simulink library "halin"  (R2021b)
settings: Solver=VariableStepAuto  StartTime=0.0  StopTime=10.0  RelTol=1e-3
undefined symbols (not defined in the file): KHAL_CAN1ABM1E2E_flg, KHAL_CAN1EPB1E2E_flg, KHAL_CAN1EPS1E2E_flg, KHAL_CAN1ESC1E2E_flg, KHAL_CAN1ESC5E2E_flg, KHAL_CAN3BMS1E2E_flg, KHAL_CAN3BMS6E2E_flg, KHAL_CAN3CCU1E2E_flg, KHAL_CAN3CCU2E2E_flg, KHAL_CAN3MCUBF1E2E_flg, KHAL_CAN3MCUBR1E2E_flg, KHAL_CAN3MCUNF1E2E_flg, KHAL_CAN3MCUNR1E2E_flg, KHAL_CAN3Shifter1E2E_flg, KHAL_CAN3Shifter2E2E_flg, KHAL_CAN6FCM2E2E_flg, KHAL_CAN6FCM4E2E_flg, TRUE
libraries: simulink x791, FVT_lib x214, hcu_lib x58
(part 17 of 25)

== system halin/HAL_IN/CAN4/ZONE_FR1 ==
  DT_CAN4_SG_ZONE_FR1 : Inport
  ChargeInletLockSta : Subsystem
  CompProEN : Subsystem
  FLTurnLPErr : Subsystem
  FLTurnLampC : Subsystem
  FLTurnLightWarning : Subsystem
  FRTurnLPErr : Subsystem
  FRTurnLampC : Subsystem
  FRTurnLightWarning : Subsystem
  FWiperAS : Subsystem
  FWiperProtection : Subsystem
  LADBHibeamIndication : Subsystem
  LADBOperationStatus : Subsystem
  LADBWarning : Subsystem
  LAHBWarning : Subsystem
  LDRLWarning : Subsystem
  LLBWarning : Subsystem
  LpositionLampWarning : Subsystem
  RADBHibeamIndication : Subsystem
  RADBOperationStatus : Subsystem
  RADBWarning : Subsystem
  RAHBWarning : Subsystem
  RDRLWarning : Subsystem
  RLBWarning : Subsystem
  RpositionLampWarning : Subsystem
  TrailerCheck : Subsystem
  TrailerModeSta : Subsystem
  ZFRBCMChargerDoorSWSta : Subsystem
  ZFRBCMHRLTurnLPNormalSta : Subsystem
  ZFRBCMHRRTurnLPHNormalSta : Subsystem
  ZFRTHCMCLEVentActYSta : Subsystem
  ZFRTHCMCREVentActYSta : Subsystem
  ZFRTHCMLEVentActYSta : Subsystem
  ZFRTHCMREVentActYSta : Subsystem
  bus_selector : BusSelector  OutputSignals=CAN4_ChargeInletLockSta
  bus_selector1 : BusSelector  OutputSignals=CAN4_CompProEN
  bus_selector10 : BusSelector  OutputSignals=CAN4_LADB_Hibeam_Indication
  bus_selector11 : BusSelector  OutputSignals=CAN4_LADB_Operation_Status
  bus_selector12 : BusSelector  OutputSignals=CAN4_LADB_Warning
  bus_selector13 : BusSelector  OutputSignals=CAN4_LAHB_Warning
  bus_selector14 : BusSelector  OutputSignals=CAN4_LDRL_Warning
  bus_selector15 : BusSelector  OutputSignals=CAN4_LLB_Warning
  bus_selector16 : BusSelector  OutputSignals=CAN4_Lposition_Lamp_Warning
  bus_selector17 : BusSelector  OutputSignals=CAN4_RADB_Hibeam_Indication
  bus_selector18 : BusSelector  OutputSignals=CAN4_RADB_Operation_Status
  bus_selector19 : BusSelector  OutputSignals=CAN4_RADB_Warning
  bus_selector2 : BusSelector  OutputSignals=CAN4_FLTurnLPErr
  bus_selector20 : BusSelector  OutputSignals=CAN4_RAHB_Warning
  bus_selector21 : BusSelector  OutputSignals=CAN4_RDRL_Warning
  bus_selector22 : BusSelector  OutputSignals=CAN4_RLB_Warning
  bus_selector23 : BusSelector  OutputSignals=CAN4_Rposition_Lamp_Warning
  bus_selector24 : BusSelector  OutputSignals=CAN4_TrailerCheck
  bus_selector25 : BusSelector  OutputSignals=CAN4_TrailerModeSta
  bus_selector26 : BusSelector  OutputSignals=CAN4_ZFR_BCM_ChargerDoorSW_Sta
  bus_selector27 : BusSelector  OutputSignals=CAN4_ZFR_BCM_HRLTurnLPNormal_Sta
  bus_selector28 : BusSelector  OutputSignals=CAN4_ZFR_BCM_HRRTurnLPHNormal_Sta
  bus_selector29 : BusSelector  OutputSignals=CAN4_ZFR_THCM_CLEVentActY_Sta
  bus_selector3 : BusSelector  OutputSignals=CAN4_FLTurnLampC
  bus_selector30 : BusSelector  OutputSignals=CAN4_ZFR_THCM_CREVentActY_Sta
  bus_selector31 : BusSelector  OutputSignals=CAN4_ZFR_THCM_LEVentActY_Sta
  bus_selector32 : BusSelector  OutputSignals=CAN4_ZFR_THCM_REVentActY_Sta
  bus_selector4 : BusSelector  OutputSignals=CAN4_FLTurn_Light_Warning
  bus_selector5 : BusSelector  OutputSignals=CAN4_FRTurnLPErr
  bus_selector6 : BusSelector  OutputSignals=CAN4_FRTurnLampC
  bus_selector7 : BusSelector  OutputSignals=CAN4_FRTurn_Light_Warning
  bus_selector8 : BusSelector  OutputSignals=CAN4_FWiperAS
  bus_selector9 : BusSelector  OutputSignals=CAN4_FWiperProtection
  VHAL_ChargeInletLockSta_flg : Outport
  VHAL_CompProEN_flg : Outport  Port=2
  VHAL_FLTurnLPErr_flg : Outport  Port=3
  VHAL_FLTurnLampC_mA : Outport  Port=4
  VHAL_FLTurnLightWarning_flg : Outport  Port=5
  VHAL_FRTurnLPErr_flg : Outport  Port=6
  VHAL_FRTurnLampC_mA : Outport  Port=7
  VHAL_FRTurnLightWarning_flg : Outport  Port=8
  VHAL_FWiperAS_flg : Outport  Port=9
  VHAL_FWiperProtection_flg : Outport  Port=10
  VHAL_LADBHibeamIndication_flg : Outport  Port=11
  VHAL_LADBOperationStatus_flg : Outport  Port=12
  VHAL_LADBWarning_flg : Outport  Port=13
  VHAL_LAHBWarning_flg : Outport  Port=14
  VHAL_LDRLWarning_flg : Outport  Port=15
  VHAL_LLBWarning_flg : Outport  Port=16
  VHAL_LpositionLampWarning_flg : Outport  Port=17
  VHAL_RADBHibeamIndication_flg : Outport  Port=18
  VHAL_RADBOperationStatus_flg : Outport  Port=19
  VHAL_RADBWarning_flg : Outport  Port=20
  VHAL_RAHBWarning_flg : Outport  Port=21
  VHAL_RDRLWarning_flg : Outport  Port=22
  VHAL_RLBWarning_flg : Outport  Port=23
  VHAL_RpositionLampWarning_flg : Outport  Port=24
  VHAL_TrailerCheck_flg : Outport  Port=25
  VHAL_TrailerModeSta_enum : Outport  Port=26
  VHAL_ZFRBCMChargerDoorSWSta_flg : Outport  Port=27
  VHAL_ZFRBCMHRLTurnLPNormalSta_flg : Outport  Port=28
  VHAL_ZFRBCMHRRTurnLPHNormalSta_flg : Outport  Port=29
  VHAL_ZFRTHCMCLEVentActYSta_pct : Outport  Port=30
  VHAL_ZFRTHCMCREVentActYSta_pct : Outport  Port=31
  VHAL_ZFRTHCMLEVentActYSta_pct : Outport  Port=32
  VHAL_ZFRTHCMREVentActYSta_pct : Outport  Port=33
  wires:
  DT_CAN4_SG_ZONE_FR1/1 -> [DT_CAN4_SG_ZONE_FR1]
  [DT_CAN4_SG_ZONE_FR1] -> bus_selector/1
  bus_selector/1 -> ChargeInletLockSta/1(ChargeInletLockSta)  "<CAN4_ChargeInletLockSta>"
  ChargeInletLockSta/1(VHAL_ChargeInletLockSta_flg) -> VHAL_ChargeInletLockSta_flg/1
  [DT_CAN4_SG_ZONE_FR1] -> bus_selector1/1
  bus_selector1/1 -> CompProEN/1(CompProEN)  "<CAN4_CompProEN>"
  CompProEN/1(VHAL_CompProEN_flg) -> VHAL_CompProEN_flg/1
  [DT_CAN4_SG_ZONE_FR1] -> bus_selector2/1
  bus_selector2/1 -> FLTurnLPErr/1(FLTurnLPErr)  "<CAN4_FLTurnLPErr>"
  FLTurnLPErr/1(VHAL_FLTurnLPErr_flg) -> VHAL_FLTurnLPErr_flg/1
  [DT_CAN4_SG_ZONE_FR1] -> bus_selector3/1
  bus_selector3/1 -> FLTurnLampC/1(FLTurnLampC)  "<CAN4_FLTurnLampC>"
  FLTurnLampC/1(VHAL_FLTurnLampC_mA) -> VHAL_FLTurnLampC_mA/1
  [DT_CAN4_SG_ZONE_FR1] -> bus_selector4/1
  bus_selector4/1 -> FLTurnLightWarning/1(FLTurn_Light_Warning)  "<CAN4_FLTurn_Light_Warning>"
  FLTurnLightWarning/1(VHAL_FLTurnLightWarning_flg) -> VHAL_FLTurnLightWarning_flg/1
  [DT_CAN4_SG_ZONE_FR1] -> bus_selector5/1
  bus_selector5/1 -> FRTurnLPErr/1(FRTurnLPErr)  "<CAN4_FRTurnLPErr>"
  FRTurnLPErr/1(VHAL_FRTurnLPErr_flg) -> VHAL_FRTurnLPErr_flg/1
  [DT_CAN4_SG_ZONE_FR1] -> bus_selector6/1
  bus_selector6/1 -> FRTurnLampC/1(FRTurnLampC)  "<CAN4_FRTurnLampC>"
  FRTurnLampC/1(VHAL_FRTurnLampC_mA) -> VHAL_FRTurnLampC_mA/1
  [DT_CAN4_SG_ZONE_FR1] -> bus_selector7/1
  bus_selector7/1 -> FRTurnLightWarning/1(FRTurn_Light_Warning)  "<CAN4_FRTurn_Light_Warning>"
  FRTurnLightWarning/1(VHAL_FRTurnLightWarning_flg) -> VHAL_FRTurnLightWarning_flg/1
  [DT_CAN4_SG_ZONE_FR1] -> bus_selector8/1
  bus_selector8/1 -> FWiperAS/1(FWiperAS)  "<CAN4_FWiperAS>"
  FWiperAS/1(VHAL_FWiperAS_flg) -> VHAL_FWiperAS_flg/1
  [DT_CAN4_SG_ZONE_FR1] -> bus_selector9/1
  bus_selector9/1 -> FWiperProtection/1(FWiperProtection)  "<CAN4_FWiperProtection>"
  FWiperProtection/1(VHAL_FWiperProtection_flg) -> VHAL_FWiperProtection_flg/1
  [DT_CAN4_SG_ZONE_FR1] -> bus_selector10/1
  bus_selector10/1 -> LADBHibeamIndication/1(LADB_Hibeam_Indication)  "<CAN4_LADB_Hibeam_Indication>"
  LADBHibeamIndication/1(VHAL_LADBHibeamIndication_flg) -> VHAL_LADBHibeamIndication_flg/1
  [DT_CAN4_SG_ZONE_FR1] -> bus_selector11/1
  bus_selector11/1 -> LADBOperationStatus/1(LADB_Operation_Status)  "<CAN4_LADB_Operation_Status>"
  LADBOperationStatus/1(VHAL_LADBOperationStatus_flg) -> VHAL_LADBOperationStatus_flg/1
  [DT_CAN4_SG_ZONE_FR1] -> bus_selector12/1
  bus_selector12/1 -> LADBWarning/1(LADB_Warning)  "<CAN4_LADB_Warning>"
  LADBWarning/1(VHAL_LADBWarning_flg) -> VHAL_LADBWarning_flg/1
  [DT_CAN4_SG_ZONE_FR1] -> bus_selector13/1
  bus_selector13/1 -> LAHBWarning/1(LAHB_Warning)  "<CAN4_LAHB_Warning>"
  LAHBWarning/1(VHAL_LAHBWarning_flg) -> VHAL_LAHBWarning_flg/1
  [DT_CAN4_SG_ZONE_FR1] -> bus_selector14/1
  bus_selector14/1 -> LDRLWarning/1(LDRL_Warning)  "<CAN4_LDRL_Warning>"
  LDRLWarning/1(VHAL_LDRLWarning_flg) -> VHAL_LDRLWarning_flg/1
  [DT_CAN4_SG_ZONE_FR1] -> bus_selector15/1
  bus_selector15/1 -> LLBWarning/1(LLB_Warning)  "<CAN4_LLB_Warning>"
  LLBWarning/1(VHAL_LLBWarning_flg) -> VHAL_LLBWarning_flg/1
  [DT_CAN4_SG_ZONE_FR1] -> bus_selector16/1
  bus_selector16/1 -> LpositionLampWarning/1(Lposition_Lamp_Warning)  "<CAN4_Lposition_Lamp_Warning>"
  LpositionLampWarning/1(VHAL_LpositionLampWarning_flg) -> VHAL_LpositionLampWarning_flg/1
  [DT_CAN4_SG_ZONE_FR1] -> bus_selector17/1
  bus_selector17/1 -> RADBHibeamIndication/1(RADB_Hibeam_Indication)  "<CAN4_RADB_Hibeam_Indication>"
  RADBHibeamIndication/1(VHAL_RADBHibeamIndication_flg) -> VHAL_RADBHibeamIndication_flg/1
  [DT_CAN4_SG_ZONE_FR1] -> bus_selector18/1
  bus_selector18/1 -> RADBOperationStatus/1(RADB_Operation_Status)  "<CAN4_RADB_Operation_Status>"
  RADBOperationStatus/1(VHAL_RADBOperationStatus_flg) -> VHAL_RADBOperationStatus_flg/1
  [DT_CAN4_SG_ZONE_FR1] -> bus_selector19/1
  bus_selector19/1 -> RADBWarning/1(RADB_Warning)  "<CAN4_RADB_Warning>"
  RADBWarning/1(VHAL_RADBWarning_flg) -> VHAL_RADBWarning_flg/1
  [DT_CAN4_SG_ZONE_FR1] -> bus_selector20/1
  bus_selector20/1 -> RAHBWarning/1(RAHB_Warning)  "<CAN4_RAHB_Warning>"
  RAHBWarning/1(VHAL_RAHBWarning_flg) -> VHAL_RAHBWarning_flg/1
  [DT_CAN4_SG_ZONE_FR1] -> bus_selector21/1
  bus_selector21/1 -> RDRLWarning/1(RDRL_Warning)  "<CAN4_RDRL_Warning>"
  RDRLWarning/1(VHAL_RDRLWarning_flg) -> VHAL_RDRLWarning_flg/1
  [DT_CAN4_SG_ZONE_FR1] -> bus_selector22/1
  bus_selector22/1 -> RLBWarning/1(RLB_Warning)  "<CAN4_RLB_Warning>"
  RLBWarning/1(VHAL_RLBWarning_flg) -> VHAL_RLBWarning_flg/1
  [DT_CAN4_SG_ZONE_FR1] -> bus_selector23/1
  bus_selector23/1 -> RpositionLampWarning/1(Rposition_Lamp_Warning)  "<CAN4_Rposition_Lamp_Warning>"
  RpositionLampWarning/1(VHAL_RpositionLampWarning_flg) -> VHAL_RpositionLampWarning_flg/1
  [DT_CAN4_SG_ZONE_FR1] -> bus_selector24/1
  bus_selector24/1 -> TrailerCheck/1(TrailerCheck)  "<CAN4_TrailerCheck>"
  TrailerCheck/1(VHAL_TrailerCheck_flg) -> VHAL_TrailerCheck_flg/1
  [DT_CAN4_SG_ZONE_FR1] -> bus_selector25/1
  bus_selector25/1 -> TrailerModeSta/1(TrailerModeSta)  "<CAN4_TrailerModeSta>"
  TrailerModeSta/1(VHAL_TrailerModeSta_enum) -> VHAL_TrailerModeSta_enum/1
  [DT_CAN4_SG_ZONE_FR1] -> bus_selector26/1
  bus_selector26/1 -> ZFRBCMChargerDoorSWSta/1(ZFR_BCM_ChargerDoorSW_Sta)  "<CAN4_ZFR_BCM_ChargerDoorSW_Sta>"
  ZFRBCMChargerDoorSWSta/1(VHAL_ZFRBCMChargerDoorSWSta_flg) -> VHAL_ZFRBCMChargerDoorSWSta_flg/1
  [DT_CAN4_SG_ZONE_FR1] -> bus_selector27/1
  bus_selector27/1 -> ZFRBCMHRLTurnLPNormalSta/1(ZFR_BCM_HRLTurnLPNormal_Sta)  "<CAN4_ZFR_BCM_HRLTurnLPNormal_Sta>"
  ZFRBCMHRLTurnLPNormalSta/1(VHAL_ZFRBCMHRLTurnLPNormalSta_flg) -> VHAL_ZFRBCMHRLTurnLPNormalSta_flg/1
  [DT_CAN4_SG_ZONE_FR1] -> bus_selector28/1
  bus_selector28/1 -> ZFRBCMHRRTurnLPHNormalSta/1(ZFR_BCM_HRRTurnLPHNormal_Sta)  "<CAN4_ZFR_BCM_HRRTurnLPHNormal_Sta>"
  ZFRBCMHRRTurnLPHNormalSta/1(VHAL_ZFRBCMHRRTurnLPHNormalSta_flg) -> VHAL_ZFRBCMHRRTurnLPHNormalSta_flg/1
  [DT_CAN4_SG_ZONE_FR1] -> bus_selector29/1
  bus_selector29/1 -> ZFRTHCMCLEVentActYSta/1(ZFR_THCM_CLEVentActY_Sta)  "<CAN4_ZFR_THCM_CLEVentActY_Sta>"
  ZFRTHCMCLEVentActYSta/1(VHAL_ZFRTHCMCLEVentActYSta_pct) -> VHAL_ZFRTHCMCLEVentActYSta_pct/1
  [DT_CAN4_SG_ZONE_FR1] -> bus_selector30/1
  bus_selector30/1 -> ZFRTHCMCREVentActYSta/1(ZFR_THCM_CREVentActY_Sta)  "<CAN4_ZFR_THCM_CREVentActY_Sta>"
  ZFRTHCMCREVentActYSta/1(VHAL_ZFRTHCMCREVentActYSta_pct) -> VHAL_ZFRTHCMCREVentActYSta_pct/1
  [DT_CAN4_SG_ZONE_FR1] -> bus_selector31/1
  bus_selector31/1 -> ZFRTHCMLEVentActYSta/1(ZFR_THCM_LEVentActY_Sta)  "<CAN4_ZFR_THCM_LEVentActY_Sta>"
  ZFRTHCMLEVentActYSta/1(VHAL_ZFRTHCMLEVentActYSta_pct) -> VHAL_ZFRTHCMLEVentActYSta_pct/1
  [DT_CAN4_SG_ZONE_FR1] -> bus_selector32/1
  bus_selector32/1 -> ZFRTHCMREVentActYSta/1(ZFR_THCM_REVentActY_Sta)  "<CAN4_ZFR_THCM_REVentActY_Sta>"
  ZFRTHCMREVentActYSta/1(VHAL_ZFRTHCMREVentActYSta_pct) -> VHAL_ZFRTHCMREVentActYSta_pct/1

== system halin/HAL_IN/CAN4/ZONE_FR_VCU ==
  DT_CAN4_SG_ZONE_FR_VCU : Inport
  AGSErr : Subsystem
  BatInTemp : Subsystem
  BatInTempErr : Subsystem
  BatOutTemp : Subsystem
  COMPErr : Subsystem
  EACProtectEnable : Subsystem
  EWP3Err : Subsystem
  EXV1Err : Subsystem
  EXV2Err : Subsystem
  FanErr : Subsystem
  FrPMMLimpHomeActReq : Subsystem
  MotorInTemp : Subsystem
  MotorInTempErr : Subsystem
  MotorOutTemp : Subsystem
  MotorOutTempErr : Subsystem
  PTHighP : Subsystem
  PTHighPErr : Subsystem
  PTHighTact : Subsystem
  PTHighTactErr : Subsystem
  PTLowP1 : Subsystem
  PTLowP1Err : Subsystem
  PTLowP2 : Subsystem
  PTLowP2Err : Subsystem
  PTLowT1 : Subsystem
  PTLowT1Err : Subsystem
  PTLowT2 : Subsystem
  PTLowT2Err : Subsystem
  SOTXVErr : Subsystem
  SOV1Err : Subsystem
  SOV2Err : Subsystem
  SOV3Err : Subsystem
  Tamb : Subsystem
  TambErr : Subsystem
  bus_selector : BusSelector  OutputSignals=CAN4_AGS_Err
  bus_selector1 : BusSelector  OutputSignals=CAN4_Bat_In_Temp
  bus_selector10 : BusSelector  OutputSignals=CAN4_FrPMMLimpHomeActReq
  bus_selector11 : BusSelector  OutputSignals=CAN4_Motor_In_Temp
  bus_selector12 : BusSelector  OutputSignals=CAN4_Motor_In_Temp_Err
  bus_selector13 : BusSelector  OutputSignals=CAN4_Motor_Out_Temp
  bus_selector14 : BusSelector  OutputSignals=CAN4_Motor_Out_Temp_Err
  bus_selector15 : BusSelector  OutputSignals=CAN4_PT_High_P
  bus_selector16 : BusSelector  OutputSignals=CAN4_PT_High_P_Err
  bus_selector17 : BusSelector  OutputSignals=CAN4_PT_High_Tact
  bus_selector18 : BusSelector  OutputSignals=CAN4_PT_High_Tact_Err
  bus_selector19 : BusSelector  OutputSignals=CAN4_PT_Low_P1
  bus_selector2 : BusSelector  OutputSignals=CAN4_Bat_In_Temp_Err
  bus_selector20 : BusSelector  OutputSignals=CAN4_PT_Low_P1_Err
  bus_selector21 : BusSelector  OutputSignals=CAN4_PT_Low_P2
  bus_selector22 : BusSelector  OutputSignals=CAN4_PT_Low_P2_Err
  bus_selector23 : BusSelector  OutputSignals=CAN4_PT_Low_T1
  bus_selector24 : BusSelector  OutputSignals=CAN4_PT_Low_T1_Err
  bus_selector25 : BusSelector  OutputSignals=CAN4_PT_Low_T2
  bus_selector26 : BusSelector  OutputSignals=CAN4_PT_Low_T2_Err
  bus_selector27 : BusSelector  OutputSignals=CAN4_SOTXV_Err
  bus_selector28 : BusSelector  OutputSignals=CAN4_SOV1_Err
  bus_selector29 : BusSelector  OutputSignals=CAN4_SOV2_Err
  bus_selector3 : BusSelector  OutputSignals=CAN4_Bat_Out_Temp
  bus_selector30 : BusSelector  OutputSignals=CAN4_SOV3_Err
  bus_selector31 : BusSelector  OutputSignals=CAN4_Tamb
  bus_selector32 : BusSelector  OutputSignals=CAN4_Tamb_Err
  bus_selector4 : BusSelector  OutputSignals=CAN4_COMP_Err
  bus_selector5 : BusSelector  OutputSignals=CAN4_EACProtectEnable
  bus_selector6 : BusSelector  OutputSignals=CAN4_EWP3_Err
  bus_selector7 : BusSelector  OutputSignals=CAN4_EXV1_Err
  bus_selector8 : BusSelector  OutputSignals=CAN4_EXV2_Err
  bus_selector9 : BusSelector  OutputSignals=CAN4_Fan_Err
  VHAL_AGSErr_enum : Outport
  VHAL_BatInTemp_C : Outport  Port=2
  VHAL_BatInTempErr_enum : Outport  Port=3
  VHAL_BatOutTemp_C : Outport  Port=4
  VHAL_COMPErr_enum : Outport  Port=5
  VHAL_EACProtectEnable_enum : Outport  Port=6
  VHAL_EWP3Err_enum : Outport  Port=7
  VHAL_EXV1Err_enum : Outport  Port=8
  VHAL_EXV2Err_enum : Outport  Port=9
  VHAL_FanErr_enum : Outport  Port=10
  VHAL_FrPMMLimpHomeActReq_flg : Outport  Port=11
  VHAL_MotorInTemp_C : Outport  Port=12
  VHAL_MotorInTempErr_enum : Outport  Port=13
  VHAL_MotorOutTemp_C : Outport  Port=14
  VHAL_MotorOutTempErr_enum : Outport  Port=15
  VHAL_PTHighP_KPa : Outport  Port=16
  VHAL_PTHighPErr_enum : Outport  Port=17
  VHAL_PTHighTact_C : Outport  Port=18
  VHAL_PTHighTactErr_enum : Outport  Port=19
  VHAL_PTLowP1_KPa : Outport  Port=20
  VHAL_PTLowP1Err_enum : Outport  Port=21
  VHAL_PTLowP2_KPa : Outport  Port=22
  VHAL_PTLowP2Err_enum : Outport  Port=23
  VHAL_PTLowT1_C : Outport  Port=24
  VHAL_PTLowT1Err_enum : Outport  Port=25
  VHAL_PTLowT2_C : Outport  Port=26
  VHAL_PTLowT2Err_enum : Outport  Port=27
  VHAL_SOTXVErr_enum : Outport  Port=28
  VHAL_SOV1Err_enum : Outport  Port=29
  VHAL_SOV2Err_enum : Outport  Port=30
  VHAL_SOV3Err_enum : Outport  Port=31
  VHAL_Tamb_C : Outport  Port=32
  VHAL_TambErr_enum : Outport  Port=33
  wires:
  DT_CAN4_SG_ZONE_FR_VCU/1 -> [DT_CAN4_SG_ZONE_FR_VCU]
  [DT_CAN4_SG_ZONE_FR_VCU] -> bus_selector/1
  bus_selector/1 -> AGSErr/1(AGS_Err)  "<CAN4_AGS_Err>"
  AGSErr/1(VHAL_AGSErr_enum) -> VHAL_AGSErr_enum/1
  [DT_CAN4_SG_ZONE_FR_VCU] -> bus_selector1/1
  bus_selector1/1 -> BatInTemp/1(Bat_In_Temp)  "<CAN4_Bat_In_Temp>"
  BatInTemp/1(VHAL_BatInTemp_C) -> VHAL_BatInTemp_C/1
  [DT_CAN4_SG_ZONE_FR_VCU] -> bus_selector2/1
  bus_selector2/1 -> BatInTempErr/1(Bat_In_Temp_Err)  "<CAN4_Bat_In_Temp_Err>"
  BatInTempErr/1(VHAL_BatInTempErr_enum) -> VHAL_BatInTempErr_enum/1
  [DT_CAN4_SG_ZONE_FR_VCU] -> bus_selector3/1
  bus_selector3/1 -> BatOutTemp/1(Bat_Out_Temp)  "<CAN4_Bat_Out_Temp>"
  BatOutTemp/1(VHAL_BatOutTemp_C) -> VHAL_BatOutTemp_C/1
  [DT_CAN4_SG_ZONE_FR_VCU] -> bus_selector4/1
  bus_selector4/1 -> COMPErr/1(COMP_Err)  "<CAN4_COMP_Err>"
  COMPErr/1(VHAL_COMPErr_enum) -> VHAL_COMPErr_enum/1
  [DT_CAN4_SG_ZONE_FR_VCU] -> bus_selector5/1
  bus_selector5/1 -> EACProtectEnable/1(EACProtectEnable)  "<CAN4_EACProtectEnable>"
  EACProtectEnable/1(VHAL_EACProtectEnable_enum) -> VHAL_EACProtectEnable_enum/1
  [DT_CAN4_SG_ZONE_FR_VCU] -> bus_selector6/1
  bus_selector6/1 -> EWP3Err/1(EWP3_Err)  "<CAN4_EWP3_Err>"
  EWP3Err/1(VHAL_EWP3Err_enum) -> VHAL_EWP3Err_enum/1
  [DT_CAN4_SG_ZONE_FR_VCU] -> bus_selector7/1
  bus_selector7/1 -> EXV1Err/1(EXV1_Err)  "<CAN4_EXV1_Err>"
  EXV1Err/1(VHAL_EXV1Err_enum) -> VHAL_EXV1Err_enum/1
  [DT_CAN4_SG_ZONE_FR_VCU] -> bus_selector8/1
  bus_selector8/1 -> EXV2Err/1(EXV2_Err)  "<CAN4_EXV2_Err>"
  EXV2Err/1(VHAL_EXV2Err_enum) -> VHAL_EXV2Err_enum/1
  [DT_CAN4_SG_ZONE_FR_VCU] -> bus_selector9/1
  bus_selector9/1 -> FanErr/1(Fan_Err)  "<CAN4_Fan_Err>"
  FanErr/1(VHAL_FanErr_enum) -> VHAL_FanErr_enum/1
  [DT_CAN4_SG_ZONE_FR_VCU] -> bus_selector10/1
  bus_selector10/1 -> FrPMMLimpHomeActReq/1(FrPMMLimpHomeActReq)  "<CAN4_FrPMMLimpHomeActReq>"
  FrPMMLimpHomeActReq/1(VHAL_FrPMMLimpHomeActReq_flg) -> VHAL_FrPMMLimpHomeActReq_flg/1
  [DT_CAN4_SG_ZONE_FR_VCU] -> bus_selector11/1
  bus_selector11/1 -> MotorInTemp/1(Motor_In_Temp)  "<CAN4_Motor_In_Temp>"
  MotorInTemp/1(VHAL_MotorInTemp_C) -> VHAL_MotorInTemp_C/1
  [DT_CAN4_SG_ZONE_FR_VCU] -> bus_selector12/1
  bus_selector12/1 -> MotorInTempErr/1(Motor_In_Temp_Err)  "<CAN4_Motor_In_Temp_Err>"
  MotorInTempErr/1(VHAL_MotorInTempErr_enum) -> VHAL_MotorInTempErr_enum/1
  [DT_CAN4_SG_ZONE_FR_VCU] -> bus_selector13/1
  bus_selector13/1 -> MotorOutTemp/1(Motor_Out_Temp)  "<CAN4_Motor_Out_Temp>"
  MotorOutTemp/1(VHAL_MotorOutTemp_C) -> VHAL_MotorOutTemp_C/1
  [DT_CAN4_SG_ZONE_FR_VCU] -> bus_selector14/1
  bus_selector14/1 -> MotorOutTempErr/1(Motor_Out_Temp_Err)  "<CAN4_Motor_Out_Temp_Err>"
  MotorOutTempErr/1(VHAL_MotorOutTempErr_enum) -> VHAL_MotorOutTempErr_enum/1
  [DT_CAN4_SG_ZONE_FR_VCU] -> bus_selector15/1
  bus_selector15/1 -> PTHighP/1(PT_High_P)  "<CAN4_PT_High_P>"
  PTHighP/1(VHAL_PTHighP_KPa) -> VHAL_PTHighP_KPa/1
  [DT_CAN4_SG_ZONE_FR_VCU] -> bus_selector16/1
  bus_selector16/1 -> PTHighPErr/1(PT_High_P_Err)  "<CAN4_PT_High_P_Err>"
  PTHighPErr/1(VHAL_PTHighPErr_enum) -> VHAL_PTHighPErr_enum/1
  [DT_CAN4_SG_ZONE_FR_VCU] -> bus_selector17/1
  bus_selector17/1 -> PTHighTact/1(PT_High_Tact)  "<CAN4_PT_High_Tact>"
  PTHighTact/1(VHAL_PTHighTact_C) -> VHAL_PTHighTact_C/1
  [DT_CAN4_SG_ZONE_FR_VCU] -> bus_selector18/1
  bus_selector18/1 -> PTHighTactErr/1(PT_High_Tact_Err)  "<CAN4_PT_High_Tact_Err>"
  PTHighTactErr/1(VHAL_PTHighTactErr_enum) -> VHAL_PTHighTactErr_enum/1
  [DT_CAN4_SG_ZONE_FR_VCU] -> bus_selector19/1
  bus_selector19/1 -> PTLowP1/1(PT_Low_P1)  "<CAN4_PT_Low_P1>"
  PTLowP1/1(VHAL_PTLowP1_KPa) -> VHAL_PTLowP1_KPa/1
  [DT_CAN4_SG_ZONE_FR_VCU] -> bus_selector20/1
  bus_selector20/1 -> PTLowP1Err/1(PT_Low_P1_Err)  "<CAN4_PT_Low_P1_Err>"
  PTLowP1Err/1(VHAL_PTLowP1Err_enum) -> VHAL_PTLowP1Err_enum/1
  [DT_CAN4_SG_ZONE_FR_VCU] -> bus_selector21/1
  bus_selector21/1 -> PTLowP2/1(PT_Low_P2)  "<CAN4_PT_Low_P2>"
  PTLowP2/1(VHAL_PTLowP2_KPa) -> VHAL_PTLowP2_KPa/1
  [DT_CAN4_SG_ZONE_FR_VCU] -> bus_selector22/1
  bus_selector22/1 -> PTLowP2Err/1(PT_Low_P2_Err)  "<CAN4_PT_Low_P2_Err>"
  PTLowP2Err/1(VHAL_PTLowP2Err_enum) -> VHAL_PTLowP2Err_enum/1
  [DT_CAN4_SG_ZONE_FR_VCU] -> bus_selector23/1
  bus_selector23/1 -> PTLowT1/1(PT_Low_T1)  "<CAN4_PT_Low_T1>"
  PTLowT1/1(VHAL_PTLowT1_C) -> VHAL_PTLowT1_C/1
  [DT_CAN4_SG_ZONE_FR_VCU] -> bus_selector24/1
  bus_selector24/1 -> PTLowT1Err/1(PT_Low_T1_Err)  "<CAN4_PT_Low_T1_Err>"
  PTLowT1Err/1(VHAL_PTLowT1Err_enum) -> VHAL_PTLowT1Err_enum/1
  [DT_CAN4_SG_ZONE_FR_VCU] -> bus_selector25/1
  bus_selector25/1 -> PTLowT2/1(PT_Low_T2)  "<CAN4_PT_Low_T2>"
  PTLowT2/1(VHAL_PTLowT2_C) -> VHAL_PTLowT2_C/1
  [DT_CAN4_SG_ZONE_FR_VCU] -> bus_selector26/1
  bus_selector26/1 -> PTLowT2Err/1(PT_Low_T2_Err)  "<CAN4_PT_Low_T2_Err>"
  PTLowT2Err/1(VHAL_PTLowT2Err_enum) -> VHAL_PTLowT2Err_enum/1
  [DT_CAN4_SG_ZONE_FR_VCU] -> bus_selector27/1
  bus_selector27/1 -> SOTXVErr/1(SOTXV_Err)  "<CAN4_SOTXV_Err>"
  SOTXVErr/1(VHAL_SOTXVErr_enum) -> VHAL_SOTXVErr_enum/1
  [DT_CAN4_SG_ZONE_FR_VCU] -> bus_selector28/1
  bus_selector28/1 -> SOV1Err/1(SOV1_Err)  "<CAN4_SOV1_Err>"
  SOV1Err/1(VHAL_SOV1Err_enum) -> VHAL_SOV1Err_enum/1
  [DT_CAN4_SG_ZONE_FR_VCU] -> bus_selector29/1
  bus_selector29/1 -> SOV2Err/1(SOV2_Err)  "<CAN4_SOV2_Err>"
  SOV2Err/1(VHAL_SOV2Err_enum) -> VHAL_SOV2Err_enum/1
  [DT_CAN4_SG_ZONE_FR_VCU] -> bus_selector30/1
  bus_selector30/1 -> SOV3Err/1(SOV3_Err)  "<CAN4_SOV3_Err>"
  SOV3Err/1(VHAL_SOV3Err_enum) -> VHAL_SOV3Err_enum/1
  [DT_CAN4_SG_ZONE_FR_VCU] -> bus_selector31/1
  bus_selector31/1 -> Tamb/1(Tamb)  "<CAN4_Tamb>"
  Tamb/1(VHAL_Tamb_C) -> VHAL_Tamb_C/1
  [DT_CAN4_SG_ZONE_FR_VCU] -> bus_selector32/1
  bus_selector32/1 -> TambErr/1(Tamb_Err)  "<CAN4_Tamb_Err>"
  TambErr/1(VHAL_TambErr_enum) -> VHAL_TambErr_enum/1

== system halin/HAL_IN/CAN4/zGW_APTC1 ==
  DT_CAN4_SG_zGW_APTC1 : Inport
  FrntPTCLeActHeatPwr : Subsystem
  FrntPTCRearLeActHeatPwr : Subsystem
  FrntPTCRearRiActHeatPwr : Subsystem
  FrntPTCRiActHeatPwr : Subsystem
  bus_selector : BusSelector  OutputSignals=CAN4_FrntPTCLeActHeatPwr
  bus_selector1 : BusSelector  OutputSignals=CAN4_FrntPTCRearLeActHeatPwr
  bus_selector2 : BusSelector  OutputSignals=CAN4_FrntPTCRearRiActHeatPwr
  bus_selector3 : BusSelector  OutputSignals=CAN4_FrntPTCRiActHeatPwr
  VHAL_FrntPTCLeActHeatPwr_W : Outport
  VHAL_FrntPTCRearLeActHeatPwr_W : Outport  Port=2
  VHAL_FrntPTCRearRiActHeatPwr_W : Outport  Port=3
  VHAL_FrntPTCRiActHeatPwr_W : Outport  Port=4
  wires:
  DT_CAN4_SG_zGW_APTC1/1 -> [DT_CAN4_SG_zGW_APTC1]
  [DT_CAN4_SG_zGW_APTC1] -> bus_selector/1
  bus_selector/1 -> FrntPTCLeActHeatPwr/1(FrntPTCLeActHeatPwr)  "<CAN4_FrntPTCLeActHeatPwr>"
  FrntPTCLeActHeatPwr/1(VHAL_FrntPTCLeActHeatPwr_W) -> VHAL_FrntPTCLeActHeatPwr_W/1
  [DT_CAN4_SG_zGW_APTC1] -> bus_selector1/1
  bus_selector1/1 -> FrntPTCRearLeActHeatPwr/1(FrntPTCRearLeActHeatPwr)  "<CAN4_FrntPTCRearLeActHeatPwr>"
  FrntPTCRearLeActHeatPwr/1(VHAL_FrntPTCRearLeActHeatPwr_W) -> VHAL_FrntPTCRearLeActHeatPwr_W/1
  [DT_CAN4_SG_zGW_APTC1] -> bus_selector2/1
  bus_selector2/1 -> FrntPTCRearRiActHeatPwr/1(FrntPTCRearRiActHeatPwr)  "<CAN4_FrntPTCRearRiActHeatPwr>"
  FrntPTCRearRiActHeatPwr/1(VHAL_FrntPTCRearRiActHeatPwr_W) -> VHAL_FrntPTCRearRiActHeatPwr_W/1
  [DT_CAN4_SG_zGW_APTC1] -> bus_selector3/1
  bus_selector3/1 -> FrntPTCRiActHeatPwr/1(FrntPTCRiActHeatPwr)  "<CAN4_FrntPTCRiActHeatPwr>"
  FrntPTCRiActHeatPwr/1(VHAL_FrntPTCRiActHeatPwr_W) -> VHAL_FrntPTCRiActHeatPwr_W/1

== system halin/HAL_IN/CAN4/zGW_CANFr1 ==
  DT_CAN4_SG_zGW_CANFr1 : Inport
  COMPActualPwr : Subsystem
  COMPConCur : Subsystem
  COMPConVolt : Subsystem
  COMPStatorSpd : Subsystem
  PTC1PowerConsumption : Subsystem
  bus_selector : BusSelector  OutputSignals=CAN4_COMP_ActualPwr
  bus_selector1 : BusSelector  OutputSignals=CAN4_COMP_ConCur
  bus_selector2 : BusSelector  OutputSignals=CAN4_COMP_ConVolt
  bus_selector3 : BusSelector  OutputSignals=CAN4_COMP_StatorSpd
  bus_selector4 : BusSelector  OutputSignals=CAN4_PTC1_PowerConsumption
  VHAL_COMPActualPwr_W : Outport
  VHAL_COMPConCur_A : Outport  Port=2
  VHAL_COMPConVolt_V : Outport  Port=3
  VHAL_COMPStatorSpd_rpm : Outport  Port=4
  VHAL_PTC1PowerConsumption_kW : Outport  Port=5
  wires:
  DT_CAN4_SG_zGW_CANFr1/1 -> [DT_CAN4_SG_zGW_CANFr1]
  [DT_CAN4_SG_zGW_CANFr1] -> bus_selector/1
  bus_selector/1 -> COMPActualPwr/1(COMP_ActualPwr)  "<CAN4_COMP_ActualPwr>"
  COMPActualPwr/1(VHAL_COMPActualPwr_W) -> VHAL_COMPActualPwr_W/1
  [DT_CAN4_SG_zGW_CANFr1] -> bus_selector1/1
  bus_selector1/1 -> COMPConCur/1(COMP_ConCur)  "<CAN4_COMP_ConCur>"
  COMPConCur/1(VHAL_COMPConCur_A) -> VHAL_COMPConCur_A/1
  [DT_CAN4_SG_zGW_CANFr1] -> bus_selector2/1
  bus_selector2/1 -> COMPConVolt/1(COMP_ConVolt)  "<CAN4_COMP_ConVolt>"
  COMPConVolt/1(VHAL_COMPConVolt_V) -> VHAL_COMPConVolt_V/1
  [DT_CAN4_SG_zGW_CANFr1] -> bus_selector3/1
  bus_selector3/1 -> COMPStatorSpd/1(COMP_StatorSpd)  "<CAN4_COMP_StatorSpd>"
  COMPStatorSpd/1(VHAL_COMPStatorSpd_rpm) -> VHAL_COMPStatorSpd_rpm/1
  [DT_CAN4_SG_zGW_CANFr1] -> bus_selector4/1
  bus_selector4/1 -> PTC1PowerConsumption/1(PTC1_PowerConsumption)  "<CAN4_PTC1_PowerConsumption>"
  PTC1PowerConsumption/1(VHAL_PTC1PowerConsumption_kW) -> VHAL_PTC1PowerConsumption_kW/1

== system halin/HAL_IN/CAN4/zGW_LINDr1 ==
  DT_CAN4_SG_zGW_LINDr1 : Inport
  CSWDimSw : Subsystem
  CSWFWasSwSta : Subsystem
  CSWFWipSwSta : Subsystem
  CSWPassSWSta : Subsystem
  CSWRWasSWSta : Subsystem
  CSWRWipIntSwSta : Subsystem
  CSWTurnSwSta : Subsystem
  FAPWL01LINResponseError : Subsystem
  LDrvMotorRelayError : Subsystem
  LDrvMotorRippleError : Subsystem
  LDrvValWdwOpened : Subsystem
  LDrvWdwPositionSts : Subsystem
  LPasMotorRelayError : Subsystem
  LPasMotorRippleError : Subsystem
  LPasValWdwOpened : Subsystem
  LPasWdwPositionSts : Subsystem
  LRLDMotorRelayError : Subsystem
  LRLDMotorRippleError : Subsystem
  LRLDValWdwOpened : Subsystem
  LRLDWdwPositionSts : Subsystem
  LRRDMotorRelayError : Subsystem
  LRRDMotorRippleError : Subsystem
  LRRDValWdwOpened : Subsystem
  LRRDWdwPositionSts : Subsystem
  RAPWL01LINResponseError : Subsystem
  RLSLampSta : Subsystem
  RLSRainSnrWiperCmd : Subsystem
  SWC2LADASSta : Subsystem
  SWC2LDriveModeSta : Subsystem
  SWC2LHomeSta : Subsystem
  SWC2LLeftSta : Subsystem
  SWC2LRegenUpSta : Subsystem
  SWC2LRightSta : Subsystem
  SWC2LScrollDownSta : Subsystem
  SWC2LScrollPressSta : Subsystem
  SWC2LScrollUpSta : Subsystem
  SWC2RCustomizeSta : Subsystem
  SWC2RLeftSta : Subsystem
  SWC2RPageSwitchSta : Subsystem
  SWC2RRegenDownSta : Subsystem
  SWC2RRightSta : Subsystem
  SWC2RScrollDownSta : Subsystem
  SWC2RScrollPressSta : Subsystem
  SWC2RScrollUpSta : Subsystem
  SWC2RVRSta : Subsystem
  SWCACCSta : Subsystem
  SWCCANCELSta : Subsystem
  SWCDistanceSta : Subsystem
  SWCDownSta : Subsystem
  SWCLKASta : Subsystem
  SWCLeftSta : Subsystem
  SWCRegenDown : Subsystem
  SWCRegenUp : Subsystem
  SWCResUpSta : Subsystem
  SWCRightSta : Subsystem
  SWCSetdownSta : Subsystem
  SWCTripSta : Subsystem
  SWCUndefinedSta : Subsystem
  SWCUpSta : Subsystem
  SWCVRSta : Subsystem
  SWCmodeSta : Subsystem
  bus_selector : BusSelector  OutputSignals=CAN4_CSW_DimSw
  bus_selector1 : BusSelector  OutputSignals=CAN4_CSW_FWasSw_Sta
  bus_selector10 : BusSelector  OutputSignals=CAN4_L_Drv_Val_Wdw_Opened
  bus_selector11 : BusSelector  OutputSignals=CAN4_L_Drv_Wdw_PositionSts
  bus_selector12 : BusSelector  OutputSignals=CAN4_L_Pas_Motor_Relay_Error
  bus_selector13 : BusSelector  OutputSignals=CAN4_L_Pas_Motor_Ripple_Error
  bus_selector14 : BusSelector  OutputSignals=CAN4_L_Pas_Val_Wdw_Opened
  bus_selector15 : BusSelector  OutputSignals=CAN4_L_Pas_Wdw_PositionSts
  bus_selector16 : BusSelector  OutputSignals=CAN4_L_RLD_Motor_Relay_Error
  bus_selector17 : BusSelector  OutputSignals=CAN4_L_RLD_Motor_Ripple_Error
  bus_selector18 : BusSelector  OutputSignals=CAN4_L_RLD_Val_Wdw_Opened
  bus_selector19 : BusSelector  OutputSignals=CAN4_L_RLD_Wdw_PositionSts
  bus_selector2 : BusSelector  OutputSignals=CAN4_CSW_FWipSw_Sta
  bus_selector20 : BusSelector  OutputSignals=CAN4_L_RRD_Motor_Relay_Error
  bus_selector21 : BusSelector  OutputSignals=CAN4_L_RRD_Motor_Ripple_Error
  bus_selector22 : BusSelector  OutputSignals=CAN4_L_RRD_Val_Wdw_Opened
  bus_selector23 : BusSelector  OutputSignals=CAN4_L_RRD_Wdw_PositionSts
  bus_selector24 : BusSelector  OutputSignals=CAN4_RAPWL_01_LIN_Response_Error
  bus_selector25 : BusSelector  OutputSignals=CAN4_RLS_Lamp_Sta
  bus_selector26 : BusSelector  OutputSignals=CAN4_RLS_RainSnrWiperCmd
  bus_selector27 : BusSelector  OutputSignals=CAN4_SWC2_L_ADAS_Sta
  bus_selector28 : BusSelector  OutputSignals=CAN4_SWC2_L_DriveMode_Sta
  bus_selector29 : BusSelector  OutputSignals=CAN4_SWC2_L_Home_Sta
  bus_selector3 : BusSelector  OutputSignals=CAN4_CSW_PassSW_Sta
  bus_selector30 : BusSelector  OutputSignals=CAN4_SWC2_L_Left_Sta
  bus_selector31 : BusSelector  OutputSignals=CAN4_SWC2_L_RegenUp_Sta
  bus_selector32 : BusSelector  OutputSignals=CAN4_SWC2_L_Right_Sta
  bus_selector33 : BusSelector  OutputSignals=CAN4_SWC2_L_ScrollDown_Sta
  bus_selector34 : BusSelector  OutputSignals=CAN4_SWC2_L_ScrollPress_Sta
  bus_selector35 : BusSelector  OutputSignals=CAN4_SWC2_L_ScrollUp_Sta
  bus_selector36 : BusSelector  OutputSignals=CAN4_SWC2_R_Customize_Sta
  bus_selector37 : BusSelector  OutputSignals=CAN4_SWC2_R_Left_Sta
  bus_selector38 : BusSelector  OutputSignals=CAN4_SWC2_R_PageSwitch_Sta
  bus_selector39 : BusSelector  OutputSignals=CAN4_SWC2_R_RegenDown_Sta
  bus_selector4 : BusSelector  OutputSignals=CAN4_CSW_RWasSW_Sta
  bus_selector40 : BusSelector  OutputSignals=CAN4_SWC2_R_Right_Sta
  bus_selector41 : BusSelector  OutputSignals=CAN4_SWC2_R_ScrollDown_Sta
  bus_selector42 : BusSelector  OutputSignals=CAN4_SWC2_R_ScrollPress_Sta
  bus_selector43 : BusSelector  OutputSignals=CAN4_SWC2_R_ScrollUp_Sta
  bus_selector44 : BusSelector  OutputSignals=CAN4_SWC2_R_VR_Sta
  bus_selector45 : BusSelector  OutputSignals=CAN4_SWC_ACC_Sta
  bus_selector46 : BusSelector  OutputSignals=CAN4_SWC_CANCEL_Sta
  bus_selector47 : BusSelector  OutputSignals=CAN4_SWC_Distance_Sta
  bus_selector48 : BusSelector  OutputSignals=CAN4_SWC_Down_Sta
  bus_selector49 : BusSelector  OutputSignals=CAN4_SWC_LKA_Sta
  bus_selector5 : BusSelector  OutputSignals=CAN4_CSW_RWipIntSw_Sta
  bus_selector50 : BusSelector  OutputSignals=CAN4_SWC_Left_Sta
  bus_selector51 : BusSelector  OutputSignals=CAN4_SWC_RegenDown
  bus_selector52 : BusSelector  OutputSignals=CAN4_SWC_RegenUp
  bus_selector53 : BusSelector  OutputSignals=CAN4_SWC_Res_Up_Sta
  bus_selector54 : BusSelector  OutputSignals=CAN4_SWC_Right_Sta
  bus_selector55 : BusSelector  OutputSignals=CAN4_SWC_Set_down_Sta
  bus_selector56 : BusSelector  OutputSignals=CAN4_SWC_Trip_Sta
  bus_selector57 : BusSelector  OutputSignals=CAN4_SWC_Undefined_Sta
  bus_selector58 : BusSelector  OutputSignals=CAN4_SWC_Up_Sta
  bus_selector59 : BusSelector  OutputSignals=CAN4_SWC_VR_Sta
  bus_selector6 : BusSelector  OutputSignals=CAN4_CSW_TurnSw_Sta
  bus_selector60 : BusSelector  OutputSignals=CAN4_SWC_mode_Sta
  bus_selector7 : BusSelector  OutputSignals=CAN4_FAPWL_01_LIN_Response_Error
  bus_selector8 : BusSelector  OutputSignals=CAN4_L_Drv_Motor_Relay_Error
  bus_selector9 : BusSelector  OutputSignals=CAN4_L_Drv_Motor_Ripple_Error
  VHAL_CSWDimSw_flg : Outport
  VHAL_CSWFWasSwSta_enum : Outport  Port=2
  VHAL_CSWFWipSwSta_enum : Outport  Port=3
  VHAL_CSWPassSWSta_flg : Outport  Port=4
  VHAL_CSWRWasSWSta_enum : Outport  Port=5
  VHAL_CSWRWipIntSwSta_enum : Outport  Port=6
  VHAL_CSWTurnSwSta_enum : Outport  Port=7
  VHAL_FAPWL01LINResponseError_flg : Outport  Port=8
  VHAL_LDrvMotorRelayError_flg : Outport  Port=9
  VHAL_LDrvMotorRippleError_flg : Outport  Port=10
  VHAL_LDrvValWdwOpened_pct : Outport  Port=11
  VHAL_LDrvWdwPositionSts_enum : Outport  Port=12
  VHAL_LPasMotorRelayError_flg : Outport  Port=13
  VHAL_LPasMotorRippleError_flg : Outport  Port=14
  VHAL_LPasValWdwOpened_pct : Outport  Port=15
  VHAL_LPasWdwPositionSts_enum : Outport  Port=16
  VHAL_LRLDMotorRelayError_flg : Outport  Port=17
  VHAL_LRLDMotorRippleError_flg : Outport  Port=18
  VHAL_LRLDValWdwOpened_pct : Outport  Port=19
  VHAL_LRLDWdwPositionSts_enum : Outport  Port=20
  VHAL_LRRDMotorRelayError_flg : Outport  Port=21
  VHAL_LRRDMotorRippleError_flg : Outport  Port=22
  VHAL_LRRDValWdwOpened_pct : Outport  Port=23
  VHAL_LRRDWdwPositionSts_enum : Outport  Port=24
  VHAL_RAPWL01LINResponseError_flg : Outport  Port=25
  VHAL_RLSLampSta_flg : Outport  Port=26
  VHAL_RLSRainSnrWiperCmd_enum : Outport  Port=27
  VHAL_SWC2LADASSta_flg : Outport  Port=28
  VHAL_SWC2LDriveModeSta_flg : Outport  Port=29
  VHAL_SWC2LHomeSta_flg : Outport  Port=30
  VHAL_SWC2LLeftSta_flg : Outport  Port=31
  VHAL_SWC2LRegenUpSta_flg : Outport  Port=32
  VHAL_SWC2LRightSta_flg : Outport  Port=33
  VHAL_SWC2LScrollDownSta_flg : Outport  Port=34
  VHAL_SWC2LScrollPressSta_flg : Outport  Port=35
  VHAL_SWC2LScrollUpSta_flg : Outport  Port=36
  VHAL_SWC2RCustomizeSta_flg : Outport  Port=37
  VHAL_SWC2RLeftSta_flg : Outport  Port=38
  VHAL_SWC2RPageSwitchSta_flg : Outport  Port=39
  VHAL_SWC2RRegenDownSta_flg : Outport  Port=40
  VHAL_SWC2RRightSta_flg : Outport  Port=41
  VHAL_SWC2RScrollDownSta_flg : Outport  Port=42
  VHAL_SWC2RScrollPressSta_flg : Outport  Port=43
  VHAL_SWC2RScrollUpSta_flg : Outport  Port=44
  VHAL_SWC2RVRSta_flg : Outport  Port=45
  VHAL_SWCACCSta_flg : Outport  Port=46
  VHAL_SWCCANCELSta_flg : Outport  Port=47
  VHAL_SWCDistanceSta_flg : Outport  Port=48
  VHAL_SWCDownSta_flg : Outport  Port=49
  VHAL_SWCLKASta_flg : Outport  Port=50
  VHAL_SWCLeftSta_flg : Outport  Port=51
  VHAL_SWCRegenDown_flg : Outport  Port=52
  VHAL_SWCRegenUp_flg : Outport  Port=53
  VHAL_SWCResUpSta_flg : Outport  Port=54
  VHAL_SWCRightSta_flg : Outport  Port=55
  VHAL_SWCSetdownSta_flg : Outport  Port=56
  VHAL_SWCTripSta_flg : Outport  Port=57
  VHAL_SWCUndefinedSta_flg : Outport  Port=58
  VHAL_SWCUpSta_flg : Outport  Port=59
  VHAL_SWCVRSta_flg : Outport  Port=60
  VHAL_SWCmodeSta_flg : Outport  Port=61
  wires:
  DT_CAN4_SG_zGW_LINDr1/1 -> [DT_CAN4_SG_zGW_LINDr1]
  [DT_CAN4_SG_zGW_LINDr1] -> bus_selector/1
  bus_selector/1 -> CSWDimSw/1(CSW_DimSw)  "<CAN4_CSW_DimSw>"
  CSWDimSw/1(VHAL_CSWDimSw_flg) -> VHAL_CSWDimSw_flg/1
  [DT_CAN4_SG_zGW_LINDr1] -> bus_selector1/1
  bus_selector1/1 -> CSWFWasSwSta/1(CSW_FWasSw_Sta)  "<CAN4_CSW_FWasSw_Sta>"
  CSWFWasSwSta/1(VHAL_CSWFWasSwSta_enum) -> VHAL_CSWFWasSwSta_enum/1
  [DT_CAN4_SG_zGW_LINDr1] -> bus_selector2/1
  bus_selector2/1 -> CSWFWipSwSta/1(CSW_FWipSw_Sta)  "<CAN4_CSW_FWipSw_Sta>"
  CSWFWipSwSta/1(VHAL_CSWFWipSwSta_enum) -> VHAL_CSWFWipSwSta_enum/1
  [DT_CAN4_SG_zGW_LINDr1] -> bus_selector3/1
  bus_selector3/1 -> CSWPassSWSta/1(CSW_PassSW_Sta)  "<CAN4_CSW_PassSW_Sta>"
  CSWPassSWSta/1(VHAL_CSWPassSWSta_flg) -> VHAL_CSWPassSWSta_flg/1
  [DT_CAN4_SG_zGW_LINDr1] -> bus_selector4/1
  bus_selector4/1 -> CSWRWasSWSta/1(CSW_RWasSW_Sta)  "<CAN4_CSW_RWasSW_Sta>"
  CSWRWasSWSta/1(VHAL_CSWRWasSWSta_enum) -> VHAL_CSWRWasSWSta_enum/1
  [DT_CAN4_SG_zGW_LINDr1] -> bus_selector5/1
  bus_selector5/1 -> CSWRWipIntSwSta/1(CSW_RWipIntSw_Sta)  "<CAN4_CSW_RWipIntSw_Sta>"
  CSWRWipIntSwSta/1(VHAL_CSWRWipIntSwSta_enum) -> VHAL_CSWRWipIntSwSta_enum/1
  [DT_CAN4_SG_zGW_LINDr1] -> bus_selector6/1
  bus_selector6/1 -> CSWTurnSwSta/1(CSW_TurnSw_Sta)  "<CAN4_CSW_TurnSw_Sta>"
  CSWTurnSwSta/1(VHAL_CSWTurnSwSta_enum) -> VHAL_CSWTurnSwSta_enum/1
  [DT_CAN4_SG_zGW_LINDr1] -> bus_selector7/1
  bus_selector7/1 -> FAPWL01LINResponseError/1(FAPWL_01_LIN_Response_Error)  "<CAN4_FAPWL_01_LIN_Response_Error>"
  FAPWL01LINResponseError/1(VHAL_FAPWL01LINResponseError_flg) -> VHAL_FAPWL01LINResponseError_flg/1
  [DT_CAN4_SG_zGW_LINDr1] -> bus_selector8/1
  bus_selector8/1 -> LDrvMotorRelayError/1(L_Drv_Motor_Relay_Error)  "<CAN4_L_Drv_Motor_Relay_Error>"
  LDrvMotorRelayError/1(VHAL_LDrvMotorRelayError_flg) -> VHAL_LDrvMotorRelayError_flg/1
  [DT_CAN4_SG_zGW_LINDr1] -> bus_selector9/1
  bus_selector9/1 -> LDrvMotorRippleError/1(L_Drv_Motor_Ripple_Error)  "<CAN4_L_Drv_Motor_Ripple_Error>"
  LDrvMotorRippleError/1(VHAL_LDrvMotorRippleError_flg) -> VHAL_LDrvMotorRippleError_flg/1
  [DT_CAN4_SG_zGW_LINDr1] -> bus_selector10/1
  bus_selector10/1 -> LDrvValWdwOpened/1(L_Drv_Val_Wdw_Opened)  "<CAN4_L_Drv_Val_Wdw_Opened>"
  LDrvValWdwOpened/1(VHAL_LDrvValWdwOpened_pct) -> VHAL_LDrvValWdwOpened_pct/1
  [DT_CAN4_SG_zGW_LINDr1] -> bus_selector11/1
  bus_selector11/1 -> LDrvWdwPositionSts/1(L_Drv_Wdw_PositionSts)  "<CAN4_L_Drv_Wdw_PositionSts>"
  LDrvWdwPositionSts/1(VHAL_LDrvWdwPositionSts_enum) -> VHAL_LDrvWdwPositionSts_enum/1
  [DT_CAN4_SG_zGW_LINDr1] -> bus_selector12/1
  bus_selector12/1 -> LPasMotorRelayError/1(L_Pas_Motor_Relay_Error)  "<CAN4_L_Pas_Motor_Relay_Error>"
  LPasMotorRelayError/1(VHAL_LPasMotorRelayError_flg) -> VHAL_LPasMotorRelayError_flg/1
  [DT_CAN4_SG_zGW_LINDr1] -> bus_selector13/1
  bus_selector13/1 -> LPasMotorRippleError/1(L_Pas_Motor_Ripple_Error)  "<CAN4_L_Pas_Motor_Ripple_Error>"
  LPasMotorRippleError/1(VHAL_LPasMotorRippleError_flg) -> VHAL_LPasMotorRippleError_flg/1
  [DT_CAN4_SG_zGW_LINDr1] -> bus_selector14/1
  bus_selector14/1 -> LPasValWdwOpened/1(L_Pas_Val_Wdw_Opened)  "<CAN4_L_Pas_Val_Wdw_Opened>"
  LPasValWdwOpened/1(VHAL_LPasValWdwOpened_pct) -> VHAL_LPasValWdwOpened_pct/1
  [DT_CAN4_SG_zGW_LINDr1] -> bus_selector15/1
  bus_selector15/1 -> LPasWdwPositionSts/1(L_Pas_Wdw_PositionSts)  "<CAN4_L_Pas_Wdw_PositionSts>"
  LPasWdwPositionSts/1(VHAL_LPasWdwPositionSts_enum) -> VHAL_LPasWdwPositionSts_enum/1
  [DT_CAN4_SG_zGW_LINDr1] -> bus_selector16/1
  bus_selector16/1 -> LRLDMotorRelayError/1(L_RLD_Motor_Relay_Error)  "<CAN4_L_RLD_Motor_Relay_Error>"
  LRLDMotorRelayError/1(VHAL_LRLDMotorRelayError_flg) -> VHAL_LRLDMotorRelayError_flg/1
  [DT_CAN4_SG_zGW_LINDr1] -> bus_selector17/1
  bus_selector17/1 -> LRLDMotorRippleError/1(L_RLD_Motor_Ripple_Error)  "<CAN4_L_RLD_Motor_Ripple_Error>"
  LRLDMotorRippleError/1(VHAL_LRLDMotorRippleError_flg) -> VHAL_LRLDMotorRippleError_flg/1
  [DT_CAN4_SG_zGW_LINDr1] -> bus_selector18/1
  bus_selector18/1 -> LRLDValWdwOpened/1(L_RLD_Val_Wdw_Opened)  "<CAN4_L_RLD_Val_Wdw_Opened>"
  LRLDValWdwOpened/1(VHAL_LRLDValWdwOpened_pct) -> VHAL_LRLDValWdwOpened_pct/1
  [DT_CAN4_SG_zGW_LINDr1] -> bus_selector19/1
  bus_selector19/1 -> LRLDWdwPositionSts/1(L_RLD_Wdw_PositionSts)  "<CAN4_L_RLD_Wdw_PositionSts>"
  LRLDWdwPositionSts/1(VHAL_LRLDWdwPositionSts_enum) -> VHAL_LRLDWdwPositionSts_enum/1
  [DT_CAN4_SG_zGW_LINDr1] -> bus_selector20/1
  bus_selector20/1 -> LRRDMotorRelayError/1(L_RRD_Motor_Relay_Error)  "<CAN4_L_RRD_Motor_Relay_Error>"
  LRRDMotorRelayError/1(VHAL_LRRDMotorRelayError_flg) -> VHAL_LRRDMotorRelayError_flg/1
  [DT_CAN4_SG_zGW_LINDr1] -> bus_selector21/1
  bus_selector21/1 -> LRRDMotorRippleError/1(L_RRD_Motor_Ripple_Error)  "<CAN4_L_RRD_Motor_Ripple_Error>"
  LRRDMotorRippleError/1(VHAL_LRRDMotorRippleError_flg) -> VHAL_LRRDMotorRippleError_flg/1
  [DT_CAN4_SG_zGW_LINDr1] -> bus_selector22/1
  bus_selector22/1 -> LRRDValWdwOpened/1(L_RRD_Val_Wdw_Opened)  "<CAN4_L_RRD_Val_Wdw_Opened>"
  LRRDValWdwOpened/1(VHAL_LRRDValWdwOpened_pct) -> VHAL_LRRDValWdwOpened_pct/1
  [DT_CAN4_SG_zGW_LINDr1] -> bus_selector23/1
  bus_selector23/1 -> LRRDWdwPositionSts/1(L_RRD_Wdw_PositionSts)  "<CAN4_L_RRD_Wdw_PositionSts>"
  LRRDWdwPositionSts/1(VHAL_LRRDWdwPositionSts_enum) -> VHAL_LRRDWdwPositionSts_enum/1
  [DT_CAN4_SG_zGW_LINDr1] -> bus_selector24/1
  bus_selector24/1 -> RAPWL01LINResponseError/1(RAPWL_01_LIN_Response_Error)  "<CAN4_RAPWL_01_LIN_Response_Error>"
  RAPWL01LINResponseError/1(VHAL_RAPWL01LINResponseError_flg) -> VHAL_RAPWL01LINResponseError_flg/1
  [DT_CAN4_SG_zGW_LINDr1] -> bus_selector25/1
  bus_selector25/1 -> RLSLampSta/1(RLS_Lamp_Sta)  "<CAN4_RLS_Lamp_Sta>"
  RLSLampSta/1(VHAL_RLSLampSta_flg) -> VHAL_RLSLampSta_flg/1
  [DT_CAN4_SG_zGW_LINDr1] -> bus_selector26/1
  bus_selector26/1 -> RLSRainSnrWiperCmd/1(RLS_RainSnrWiperCmd)  "<CAN4_RLS_RainSnrWiperCmd>"
  RLSRainSnrWiperCmd/1(VHAL_RLSRainSnrWiperCmd_enum) -> VHAL_RLSRainSnrWiperCmd_enum/1
  [DT_CAN4_SG_zGW_LINDr1] -> bus_selector27/1
  bus_selector27/1 -> SWC2LADASSta/1(SWC2_L_ADAS_Sta)  "<CAN4_SWC2_L_ADAS_Sta>"
  SWC2LADASSta/1(VHAL_SWC2LADASSta_flg) -> VHAL_SWC2LADASSta_flg/1
  [DT_CAN4_SG_zGW_LINDr1] -> bus_selector28/1
  bus_selector28/1 -> SWC2LDriveModeSta/1(SWC2_L_DriveMode_Sta)  "<CAN4_SWC2_L_DriveMode_Sta>"
  SWC2LDriveModeSta/1(VHAL_SWC2LDriveModeSta_flg) -> VHAL_SWC2LDriveModeSta_flg/1
  [DT_CAN4_SG_zGW_LINDr1] -> bus_selector29/1
  bus_selector29/1 -> SWC2LHomeSta/1(SWC2_L_Home_Sta)  "<CAN4_SWC2_L_Home_Sta>"
  SWC2LHomeSta/1(VHAL_SWC2LHomeSta_flg) -> VHAL_SWC2LHomeSta_flg/1
  [DT_CAN4_SG_zGW_LINDr1] -> bus_selector30/1
  bus_selector30/1 -> SWC2LLeftSta/1(SWC2_L_Left_Sta)  "<CAN4_SWC2_L_Left_Sta>"
  SWC2LLeftSta/1(VHAL_SWC2LLeftSta_flg) -> VHAL_SWC2LLeftSta_flg/1
  [DT_CAN4_SG_zGW_LINDr1] -> bus_selector31/1
  bus_selector31/1 -> SWC2LRegenUpSta/1(SWC2_L_RegenUp_Sta)  "<CAN4_SWC2_L_RegenUp_Sta>"
  SWC2LRegenUpSta/1(VHAL_SWC2LRegenUpSta_flg) -> VHAL_SWC2LRegenUpSta_flg/1
  [DT_CAN4_SG_zGW_LINDr1] -> bus_selector32/1
  bus_selector32/1 -> SWC2LRightSta/1(SWC2_L_Right_Sta)  "<CAN4_SWC2_L_Right_Sta>"
  SWC2LRightSta/1(VHAL_SWC2LRightSta_flg) -> VHAL_SWC2LRightSta_flg/1
  [DT_CAN4_SG_zGW_LINDr1] -> bus_selector33/1
  bus_selector33/1 -> SWC2LScrollDownSta/1(SWC2_L_ScrollDown_Sta)  "<CAN4_SWC2_L_ScrollDown_Sta>"
  SWC2LScrollDownSta/1(VHAL_SWC2LScrollDownSta_flg) -> VHAL_SWC2LScrollDownSta_flg/1
  [DT_CAN4_SG_zGW_LINDr1] -> bus_selector34/1
  bus_selector34/1 -> SWC2LScrollPressSta/1(SWC2_L_ScrollPress_Sta)  "<CAN4_SWC2_L_ScrollPress_Sta>"
  SWC2LScrollPressSta/1(VHAL_SWC2LScrollPressSta_flg) -> VHAL_SWC2LScrollPressSta_flg/1
  [DT_CAN4_SG_zGW_LINDr1] -> bus_selector35/1
  bus_selector35/1 -> SWC2LScrollUpSta/1(SWC2_L_ScrollUp_Sta)  "<CAN4_SWC2_L_ScrollUp_Sta>"
  SWC2LScrollUpSta/1(VHAL_SWC2LScrollUpSta_flg) -> VHAL_SWC2LScrollUpSta_flg/1
  [DT_CAN4_SG_zGW_LINDr1] -> bus_selector36/1
  bus_selector36/1 -> SWC2RCustomizeSta/1(SWC2_R_Customize_Sta)  "<CAN4_SWC2_R_Customize_Sta>"
  SWC2RCustomizeSta/1(VHAL_SWC2RCustomizeSta_flg) -> VHAL_SWC2RCustomizeSta_flg/1
  [DT_CAN4_SG_zGW_LINDr1] -> bus_selector37/1
  bus_selector37/1 -> SWC2RLeftSta/1(SWC2_R_Left_Sta)  "<CAN4_SWC2_R_Left_Sta>"
  SWC2RLeftSta/1(VHAL_SWC2RLeftSta_flg) -> VHAL_SWC2RLeftSta_flg/1
  [DT_CAN4_SG_zGW_LINDr1] -> bus_selector38/1
  bus_selector38/1 -> SWC2RPageSwitchSta/1(SWC2_R_PageSwitch_Sta)  "<CAN4_SWC2_R_PageSwitch_Sta>"
  SWC2RPageSwitchSta/1(VHAL_SWC2RPageSwitchSta_flg) -> VHAL_SWC2RPageSwitchSta_flg/1
  [DT_CAN4_SG_zGW_LINDr1] -> bus_selector39/1
  bus_selector39/1 -> SWC2RRegenDownSta/1(SWC2_R_RegenDown_Sta)  "<CAN4_SWC2_R_RegenDown_Sta>"
  SWC2RRegenDownSta/1(VHAL_SWC2RRegenDownSta_flg) -> VHAL_SWC2RRegenDownSta_flg/1
  [DT_CAN4_SG_zGW_LINDr1] -> bus_selector40/1
  bus_selector40/1 -> SWC2RRightSta/1(SWC2_R_Right_Sta)  "<CAN4_SWC2_R_Right_Sta>"
  SWC2RRightSta/1(VHAL_SWC2RRightSta_flg) -> VHAL_SWC2RRightSta_flg/1
  [DT_CAN4_SG_zGW_LINDr1] -> bus_selector41/1
  bus_selector41/1 -> SWC2RScrollDownSta/1(SWC2_R_ScrollDown_Sta)  "<CAN4_SWC2_R_ScrollDown_Sta>"
  SWC2RScrollDownSta/1(VHAL_SWC2RScrollDownSta_flg) -> VHAL_SWC2RScrollDownSta_flg/1
  [DT_CAN4_SG_zGW_LINDr1] -> bus_selector42/1
  bus_selector42/1 -> SWC2RScrollPressSta/1(SWC2_R_ScrollPress_Sta)  "<CAN4_SWC2_R_ScrollPress_Sta>"
  SWC2RScrollPressSta/1(VHAL_SWC2RScrollPressSta_flg) -> VHAL_SWC2RScrollPressSta_flg/1
  [DT_CAN4_SG_zGW_LINDr1] -> bus_selector43/1
  bus_selector43/1 -> SWC2RScrollUpSta/1(SWC2_R_ScrollUp_Sta)  "<CAN4_SWC2_R_ScrollUp_Sta>"
  SWC2RScrollUpSta/1(VHAL_SWC2RScrollUpSta_flg) -> VHAL_SWC2RScrollUpSta_flg/1
  [DT_CAN4_SG_zGW_LINDr1] -> bus_selector44/1
  bus_selector44/1 -> SWC2RVRSta/1(SWC2_R_VR_Sta)  "<CAN4_SWC2_R_VR_Sta>"
  SWC2RVRSta/1(VHAL_SWC2RVRSta_flg) -> VHAL_SWC2RVRSta_flg/1
  [DT_CAN4_SG_zGW_LINDr1] -> bus_selector45/1
  bus_selector45/1 -> SWCACCSta/1(SWC_ACC_Sta)  "<CAN4_SWC_ACC_Sta>"
  SWCACCSta/1(VHAL_SWCACCSta_flg) -> VHAL_SWCACCSta_flg/1
  [DT_CAN4_SG_zGW_LINDr1] -> bus_selector46/1
  bus_selector46/1 -> SWCCANCELSta/1(SWC_CANCEL_Sta)  "<CAN4_SWC_CANCEL_Sta>"
  SWCCANCELSta/1(VHAL_SWCCANCELSta_flg) -> VHAL_SWCCANCELSta_flg/1
  [DT_CAN4_SG_zGW_LINDr1] -> bus_selector47/1
  bus_selector47/1 -> SWCDistanceSta/1(SWC_Distance_Sta)  "<CAN4_SWC_Distance_Sta>"
  SWCDistanceSta/1(VHAL_SWCDistanceSta_flg) -> VHAL_SWCDistanceSta_flg/1
  [DT_CAN4_SG_zGW_LINDr1] -> bus_selector48/1
  bus_selector48/1 -> SWCDownSta/1(SWC_Down_Sta)  "<CAN4_SWC_Down_Sta>"
  SWCDownSta/1(VHAL_SWCDownSta_flg) -> VHAL_SWCDownSta_flg/1
  [DT_CAN4_SG_zGW_LINDr1] -> bus_selector49/1
  bus_selector49/1 -> SWCLKASta/1(SWC_LKA_Sta)  "<CAN4_SWC_LKA_Sta>"
  SWCLKASta/1(VHAL_SWCLKASta_flg) -> VHAL_SWCLKASta_flg/1
  [DT_CAN4_SG_zGW_LINDr1] -> bus_selector50/1
  bus_selector50/1 -> SWCLeftSta/1(SWC_Left_Sta)  "<CAN4_SWC_Left_Sta>"
  SWCLeftSta/1(VHAL_SWCLeftSta_flg) -> VHAL_SWCLeftSta_flg/1
  [DT_CAN4_SG_zGW_LINDr1] -> bus_selector51/1
  bus_selector51/1 -> SWCRegenDown/1(SWC_RegenDown)  "<CAN4_SWC_RegenDown>"
  SWCRegenDown/1(VHAL_SWCRegenDown_flg) -> VHAL_SWCRegenDown_flg/1
  [DT_CAN4_SG_zGW_LINDr1] -> bus_selector52/1
  bus_selector52/1 -> SWCRegenUp/1(SWC_RegenUp)  "<CAN4_SWC_RegenUp>"
  SWCRegenUp/1(VHAL_SWCRegenUp_flg) -> VHAL_SWCRegenUp_flg/1
  [DT_CAN4_SG_zGW_LINDr1] -> bus_selector53/1
  bus_selector53/1 -> SWCResUpSta/1(SWC_Res_Up_Sta)  "<CAN4_SWC_Res_Up_Sta>"
  SWCResUpSta/1(VHAL_SWCResUpSta_flg) -> VHAL_SWCResUpSta_flg/1
  [DT_CAN4_SG_zGW_LINDr1] -> bus_selector54/1
  bus_selector54/1 -> SWCRightSta/1(SWC_Right_Sta)  "<CAN4_SWC_Right_Sta>"
  SWCRightSta/1(VHAL_SWCRightSta_flg) -> VHAL_SWCRightSta_flg/1
  [DT_CAN4_SG_zGW_LINDr1] -> bus_selector55/1
  bus_selector55/1 -> SWCSetdownSta/1(SWC_Set_down_Sta)  "<CAN4_SWC_Set_down_Sta>"
  SWCSetdownSta/1(VHAL_SWCSetdownSta_flg) -> VHAL_SWCSetdownSta_flg/1
  [DT_CAN4_SG_zGW_LINDr1] -> bus_selector56/1
  bus_selector56/1 -> SWCTripSta/1(SWC_Trip_Sta)  "<CAN4_SWC_Trip_Sta>"
  SWCTripSta/1(VHAL_SWCTripSta_flg) -> VHAL_SWCTripSta_flg/1
  [DT_CAN4_SG_zGW_LINDr1] -> bus_selector57/1
  bus_selector57/1 -> SWCUndefinedSta/1(SWC_Undefined_Sta)  "<CAN4_SWC_Undefined_Sta>"
  SWCUndefinedSta/1(VHAL_SWCUndefinedSta_flg) -> VHAL_SWCUndefinedSta_flg/1
  [DT_CAN4_SG_zGW_LINDr1] -> bus_selector58/1
  bus_selector58/1 -> SWCUpSta/1(SWC_Up_Sta)  "<CAN4_SWC_Up_Sta>"
  SWCUpSta/1(VHAL_SWCUpSta_flg) -> VHAL_SWCUpSta_flg/1
  [DT_CAN4_SG_zGW_LINDr1] -> bus_selector59/1
  bus_selector59/1 -> SWCVRSta/1(SWC_VR_Sta)  "<CAN4_SWC_VR_Sta>"
  SWCVRSta/1(VHAL_SWCVRSta_flg) -> VHAL_SWCVRSta_flg/1
  [DT_CAN4_SG_zGW_LINDr1] -> bus_selector60/1
  bus_selector60/1 -> SWCmodeSta/1(SWC_mode_Sta)  "<CAN4_SWC_mode_Sta>"
  SWCmodeSta/1(VHAL_SWCmodeSta_flg) -> VHAL_SWCmodeSta_flg/1

== system halin/HAL_IN/CAN4/zGW_LINDr2 ==
  DT_CAN4_SG_zGW_LINDr2 : Inport
  ACT1ResponseError : Subsystem
  bus_selector : BusSelector  OutputSignals=CAN4_ACT1_Response_Error
  VHAL_ACT1ResponseError_flg : Outport
  wires:
  DT_CAN4_SG_zGW_LINDr2/1 -> [DT_CAN4_SG_zGW_LINDr2]
  [DT_CAN4_SG_zGW_LINDr2] -> bus_selector/1
  bus_selector/1 -> ACT1ResponseError/1(ACT1_Response_Error)  "<CAN4_ACT1_Response_Error>"
  ACT1ResponseError/1(VHAL_ACT1ResponseError_flg) -> VHAL_ACT1ResponseError_flg/1

== system halin/HAL_IN/CAN4/zGW_LINFr1 ==
  DT_CAN4_SG_zGW_LINFr1 : Inport
  AGSActualPosition : Subsystem
  FGSIntenRspSta : Subsystem
  bus_selector : BusSelector  OutputSignals=CAN4_AGS_Actual_Position
  bus_selector1 : BusSelector  OutputSignals=CAN4_FGS_IntenRsp_Sta
  VHAL_AGSActualPosition_enum : Outport
  VHAL_FGSIntenRspSta_enum : Outport  Port=2
  wires:
  DT_CAN4_SG_zGW_LINFr1/1 -> [DT_CAN4_SG_zGW_LINFr1]
  [DT_CAN4_SG_zGW_LINFr1] -> bus_selector/1
  bus_selector/1 -> AGSActualPosition/1(AGS_Actual_Position)  "<CAN4_AGS_Actual_Position>"
  AGSActualPosition/1(VHAL_AGSActualPosition_enum) -> VHAL_AGSActualPosition_enum/1
  [DT_CAN4_SG_zGW_LINFr1] -> bus_selector1/1
  bus_selector1/1 -> FGSIntenRspSta/1(FGS_IntenRsp_Sta)  "<CAN4_FGS_IntenRsp_Sta>"
  FGSIntenRspSta/1(VHAL_FGSIntenRspSta_enum) -> VHAL_FGSIntenRspSta_enum/1
